simulink model "magball"  (Simulink 6.0)
settings: Solver=ode45  StartTime=0.0  StopTime=10  RelTol=1e-3
PreLoadFcn:
  | magballdat
undefined symbols (not defined in the file or in its folder): beta, L, m, R
settings Model: Creator=lparsons  LastModifiedBy=lparsons  BufferReuse=off
settings DataIOCC: InitialState=x0  SignalLoggingName=logsOut
settings OptimizationCC: BlockReduction=off  InlineParams=on  BufferReuse=off  MultiInstanced=off
settings FormatCC: IgnoreBidirectionalLines=off
settings HardwareCC: TargetUnknown=on
settings CodeAppCC: FileBanners=off  CustomSymbols=off
settings GRTTargetCC: TargetFcnLib=iso_c_tmw.mat  IsERTTarget=off

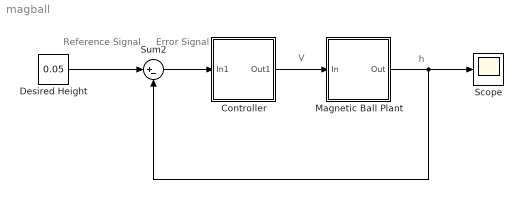
== system magball ==
  note: Error
      | Signal
  note: Reference
      | Signal
  note: V
  note: h
  Controller : Subsystem
  Desired Height : Constant  Value=0.05
  Magnetic Ball Plant : Subsystem
  Scope : Scope
  Sum2 : Sum  Inputs=|+-
  wires:
  Magnetic Ball Plant/1(Out) -> Scope/1, Sum2/2
  Sum2/1 -> Controller/1(In1)
  Controller/1(Out1) -> Magnetic Ball Plant/1(In)
  Desired Height/1 -> Sum2/1

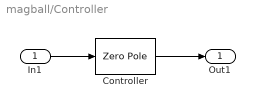
== system magball/Controller ==
  In1 : Inport
  Controller : ZeroPole  Zeros=[-11.5000+5.7900i,-11.5000-5.7900i]  Poles=[0 -1000]  Gain=-3.3057e+004
  Out1 : Outport
  wires:
  In1/1 -> Controller/1
  Controller/1 -> Out1/1

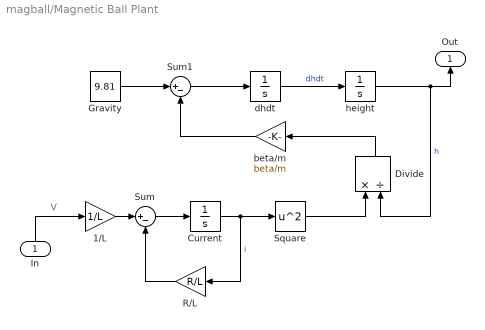
== system magball/Magnetic Ball Plant ==
  note: V
  In : Inport  Orientation=up
  1/L : Gain  Gain=1/L
  Current : Integrator  InitialCondition=7.0036
  Divide : Product  Orientation=up  Inputs=*/  OutScaling=2^-10
  Gravity : Constant  Value=9.81
  R/L : Gain  Orientation=left  Gain=R/L
  Square : Math  Operator=square  SaturateOnIntegerOverflow=on
  Sum : Sum  Inputs=|+-
  Sum1 : Sum  Inputs=|+-
  beta/m : Gain  Orientation=left  Gain=beta/m
  dhdt : Integrator
  height : Integrator  InitialCondition=0.05
  Out : Outport  Orientation=up
  wires:
  dhdt/1 -> height/1  "dhdt"
  height/1 -> Out/1, Divide/2  "h"
  Sum/1 -> Current/1
  1/L/1 -> Sum/1
  R/L/1 -> Sum/2
  Current/1 -> Square/1, R/L/1  "i"
  Square/1 -> Divide/1
  Divide/1 -> beta/m/1
  Gravity/1 -> Sum1/1
  beta/m/1 -> Sum1/2
  Sum1/1 -> dhdt/1
  In/1 -> 1/L/1
